simulink model "sampleModel25"  (R2021b)
settings: Solver=VariableStepAuto  StartTime=0.0  StopTime=10.0  RelTol=1e-3
undefined symbols (not defined in the file or in its folder): DiscIntNeverNeededParam, Newton, Raphson
libraries: simulink x8, slpidlib x1
settings Model: Creator=user  LastModifiedBy=user

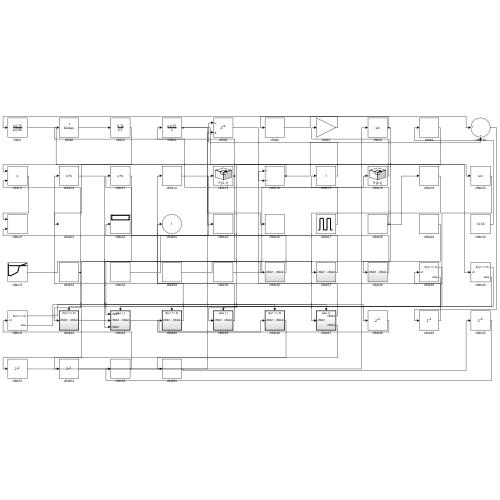
[thumbnail: Simulink's stored preview of the top-level diagram]
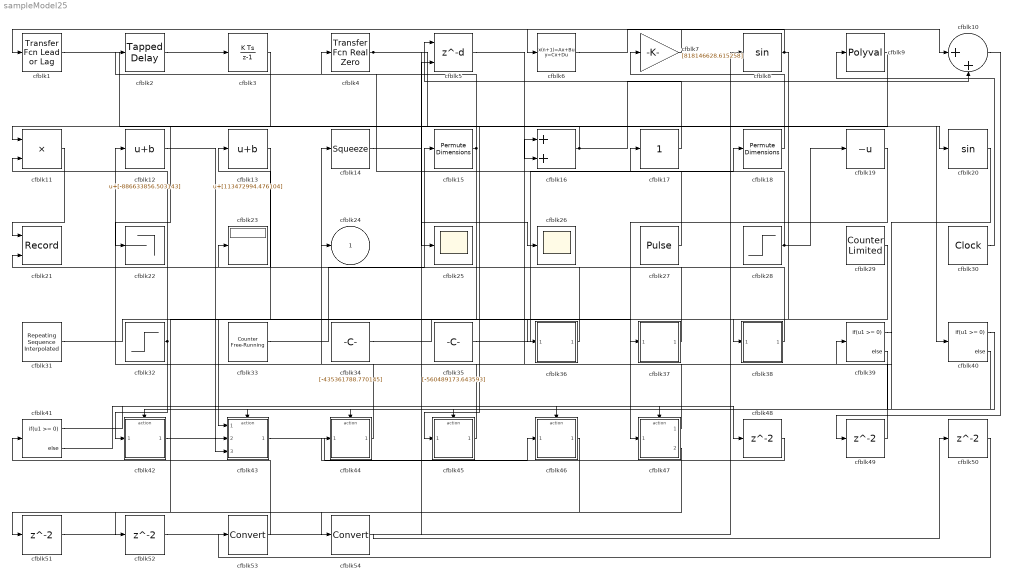
== system sampleModel25 ==
  cfblk1 : simulink/Discrete/Transfer Fcn Lead or Lag  PoleZ=0.95  ZeroZ=0.75  ICPrevOutput=0.0  ICPrevInput=0.0  DoSatur=off
      settings: SourceProductBaseCode=SL
  cfblk10 : Sum  Inputs=|++
  cfblk11 : Product  Inputs=**
  cfblk12 : Bias  Bias=[-886633856.503143]
  cfblk13 : Bias  Bias=[113472994.476104]
  cfblk14 : Squeeze
  cfblk15 : PermuteDimensions
  cfblk16 : Sum
  cfblk17 : simulink/Math Operations/Slider Gain  gain=1  low=0  high=2
  cfblk18 : PermuteDimensions
  cfblk19 : UnaryMinus
  cfblk2 : simulink/Discrete/Tapped Delay  vinit=0.0  samptime=-1  NumDelays=1  DelayOrder=Oldest  includeCurrent=off
  cfblk20 : Trigonometry
  cfblk21 : Record  FileSettingsInternal="{\"entries\":[{\"content\":{\"excelSettings\":{\"content\":{},\"type\":\"Streamout.ExcelSettings\"}},\"type\":\"Streamout.FileSettingStorage\",\"uuid\":\"81ea7c7e-9fea-4c93-8eb7-3e8b3ac382b8\"}],\"packageUris\":[\"http://schema.mathworks.com/mf0/streamout_blocks/R2020a\"],\"version\":\"1.0\"}"  Layout=[1 1]  SignalsInternal="{\"entries\":[{\"content\":{\"signals\":[{\"content\":{\"blockPath\":[\"sampleModel25/cfblk21\"],\"channel\":[],\"dimensions\":[1],\"domain\":\"sampleModel25/cfblk21\",\"lineColor\":\"#a2142f\",\"plots\":[1],\"port\":1,\"sid\":[\"\"],\"signalID\":958,\"signalName\":\"cfblk11\"},\"type\":\"RecordBlkView.Signal\",\"uuid\":\"227c1af8-843d-4dbb-83c8-0e7a03416cd8\"},{\"content\":{\"blockPath\":[\"sampleModel25/cfblk21\"],\"channel\":[],\"dimensions\":[1],\"domain\":\"sampleModel25/cfblk21\",\"lineColor\":\"#139fff\",\"plots\":[1],\"port\":2,\"sid\":[\"\"],\"signalID\":962,\"signalName\":\"cfblk36\"},\"type\":\"RecordBlkView.Signal\",\"uuid\":\"4e12becd-70fb-4f71-8634-a0132a2030ff\"}]},\"type\":\"RecordBlkView.InputSignals\",\"uuid\":\"b961e02f-62d7-4da1-8324-0dc8cbebac20\"}],\"packageUris\":[\"http://schema.mathworks.com/mf0/streamout_blocks/R2020a\"],\"version\":\"1.0\"}"  VisualizationBindings="{\"xyplotplugin\":{\"info\":[{\"series\":[{\"bindingParametersList\":[{\"parameter\":\"X-Axis\",\"signalID\":958,\"signalName\":\"cfblk11\"},{\"parameter\":\"Y-Axis\",\"signalID\":962,\"signalName\":\"cfblk36\"}],\"seriesID\":47306}],\"subplotID\":1}]}}"  CompatibilityTag=XY
  cfblk22 : Terminator
  cfblk23 : Display
  cfblk25 : Scope
  cfblk26 : Scope
  cfblk27 : DiscretePulseGenerator  PulseType=Time based  Amplitude=[-185017419.395854]  Period=[23344587.836266]  PulseWidth=5  PhaseDelay=[5.000000]
  cfblk28 : Step  Time=[16.000000]  Before=[417268794.168945]  After=[174121089.074614]  SampleTime=0
  cfblk29 : simulink/Sources/Counter Limited  uplimit=[239.000000]  tsamp=-1
  cfblk3 : DiscreteIntegrator  ICPrevOutput=DiscIntNeverNeededParam  ICPrevScaledInput=DiscIntNeverNeededParam
  cfblk30 : DigitalClock
  cfblk31 : simulink/Sources/Repeating Sequence Interpolated  OutValues=[-871882158.098314, -993261613.147159, -621854313.016368, -17592622.938083, 232937701.934326]  TimeValues=[0 0.1 0.5 0.6 1].'  LookUpMeth=Interpolation-Use End Values  tsamp=0.01  OutMin=[]  OutMax=[]  OutDataTypeStr=double  OutputDataTypeScalingMode=double  OutDataType=fixdt(0,8)  OutScaling=2^-10
  cfblk32 : Step  Time=[7.000000]  Before=[-371638337.003964]  After=[-824289697.887476]  SampleTime=0
  cfblk33 : simulink/Sources/Counter Free-Running  NumBits=[25.000000]  tsamp=-1
  cfblk34 : Constant  Value=[-435361788.770145]  SampleTime=1
  cfblk35 : Constant  Value=[-560489173.643593]  SampleTime=1
  cfblk36 : Subsystem
  cfblk37 : Subsystem
  cfblk38 : Subsystem
  cfblk39 : If  IfExpression=u1 >= 0  SampleTime=1
  cfblk4 : simulink/Discrete/Transfer Fcn Real Zero  ZeroZ=0.75  ICPrevInput=0.0  DoSatur=off
      settings: SourceProductBaseCode=SL
  cfblk40 : If  IfExpression=u1 >= 0  SampleTime=1
  cfblk41 : If  IfExpression=u1 >= 0  SampleTime=1
  cfblk42 : Subsystem  TreatAsAtomicUnit=on
  cfblk43 : Subsystem  TreatAsAtomicUnit=on
  cfblk44 : Subsystem  TreatAsAtomicUnit=on
  cfblk45 : Subsystem  TreatAsAtomicUnit=on
  cfblk46 : Subsystem  TreatAsAtomicUnit=on
  cfblk47 : Subsystem  TreatAsAtomicUnit=on
  cfblk{48..52} (5 alike) : Delay  SampleTime=1
  cfblk5 : Delay  DelayLengthSource=Input port  SampleTime=1
      settings: InputPortMap=u0,p1
  cfblk53 : DataTypeConversion
  cfblk54 : DataTypeConversion
  cfblk6 : DiscreteStateSpace
  cfblk7 : Gain  Gain=[818146628.615258]
  cfblk8 : Trigonometry
  cfblk9 : Polyval  Coefs=[ +2.081618890e-019, -1.441693666e-014, +4.719686976e-010, -8.536869453e-006, +1.621573104e-001, -8.087801117e+001 ]
  cfblk24 : Outport
  wires:
  cfblk29/1 -> cfblk43/1(cfblk1)
  cfblk32/1 -> cfblk42/1(cfblk1), cfblk11/2
  cfblk20/1 -> cfblk39/1
  cfblk8/1 -> cfblk1/1, cfblk38/1(cfblk1)
  cfblk28/1 -> cfblk17/1, cfblk19/1
  cfblk33/1 -> cfblk15/1
  cfblk37/1(cfblk2) -> cfblk23/1
  cfblk18/1 -> cfblk7/1
  cfblk47/1(cfblk2) -> cfblk14/1
  cfblk43/1(cfblk2) -> cfblk46/1(cfblk1)
  cfblk35/1 -> cfblk18/1
  cfblk17/1 -> cfblk5/1
  cfblk44/1(cfblk2) -> cfblk12/1
  cfblk7/1 -> cfblk6/1
  cfblk3/1 -> cfblk22/1
  cfblk30/1 -> cfblk9/1
  cfblk27/1 -> cfblk4/1
  cfblk15/1 -> cfblk43/2(cfblk4), cfblk2/1
  cfblk38/1(cfblk2) -> cfblk13/1
  cfblk19/1 -> cfblk47/1(cfblk1)
  cfblk11/1 -> cfblk21/1
  cfblk45/1(cfblk2) -> cfblk24/1
  cfblk31/1 -> cfblk37/1(cfblk1)
  cfblk2/1 -> cfblk3/1
  cfblk14/1 -> cfblk26/1
  cfblk1/1 -> cfblk25/1
  cfblk34/1 -> cfblk36/1(cfblk1)
  cfblk5/1 -> cfblk20/1
  cfblk16/1 -> cfblk11/1, cfblk10/2
  cfblk6/1 -> cfblk10/1
  cfblk4/1 -> cfblk40/1, cfblk16/2
  cfblk36/1(cfblk2) -> cfblk21/2
  cfblk9/1 -> cfblk45/1(cfblk1)
  cfblk42/1(cfblk2) -> cfblk43/3(cfblk5)
  cfblk39/1 -> cfblk42/Action
  cfblk39/2 -> cfblk43/Action
  cfblk40/1 -> cfblk44/Action
  cfblk40/2 -> cfblk45/Action
  cfblk41/1 -> cfblk46/Action
  cfblk41/2 -> cfblk47/Action
  cfblk12/1 -> cfblk48/1
  cfblk48/1 -> cfblk44/1(cfblk1)
  cfblk10/1 -> cfblk49/1
  cfblk49/1 -> cfblk16/1
  cfblk47/2(cfblk4) -> cfblk51/1
  cfblk51/1 -> cfblk5/2
  cfblk13/1 -> cfblk52/1
  cfblk52/1 -> cfblk8/1
  cfblk50/1 -> cfblk53/1
  cfblk53/1 -> cfblk41/1
  cfblk46/1(cfblk2) -> cfblk54/1
  cfblk54/1 -> cfblk50/1

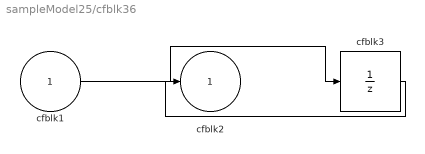
== system sampleModel25/cfblk36 ==
  cfblk1 : Inport
  cfblk3 : UnitDelay  HasFrameUpgradeWarning=on
  cfblk2 : Outport
  wires:
  cfblk1/1 -> cfblk3/1
  cfblk3/1 -> cfblk2/1

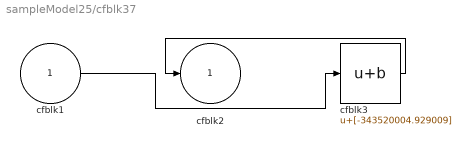
== system sampleModel25/cfblk37 ==
  cfblk1 : Inport
  cfblk3 : Bias  Bias=[-343520004.929009]
  cfblk2 : Outport
  wires:
  cfblk3/1 -> cfblk2/1
  cfblk1/1 -> cfblk3/1

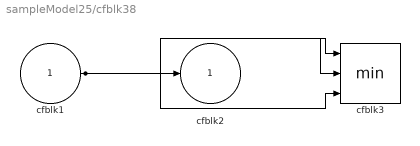
== system sampleModel25/cfblk38 ==
  cfblk1 : Inport
  cfblk3 : MinMax  Inputs=3
  cfblk2 : Outport
  wires:
  cfblk1/1 -> cfblk2/1, cfblk3/1, cfblk3/2, cfblk3/3

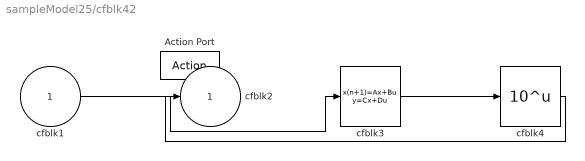
== system sampleModel25/cfblk42 ==
  cfblk1 : Inport
  Action Port : ActionPort  ActionPortLabel=if(u1 >= 0)
  cfblk3 : DiscreteStateSpace  SampleTime=-1
  cfblk4 : Math  Operator=10^u  SaturateOnIntegerOverflow=on
  cfblk2 : Outport
  wires:
  cfblk1/1 -> cfblk3/1
  cfblk3/1 -> cfblk4/1
  cfblk4/1 -> cfblk2/1

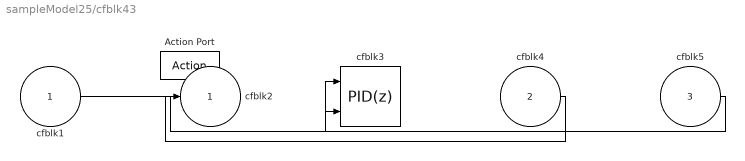
== system sampleModel25/cfblk43 ==
  cfblk1 : Inport
  cfblk4 : Inport  Port=2
  cfblk5 : Inport  Port=3
  Action Port : ActionPort  ActionPortLabel=else
  cfblk3 : slpidlib/PID Controller (2DOF)  Controller=PID  Form=Parallel  TimeDomain=Discrete-time  UseExternalTs=off  SampleTime=-1  IntegratorMethod=Forward Euler  FilterMethod=Forward Euler  ControllerParametersSource=internal  P=1  I=1  D=0  UseFilter=on  N=100  b=1  c=1  TunerSelectOption=Transfer Function Based (PID Tuner App)  InitialConditionSource=internal  InitialConditionForIntegrator=0  InitialConditionForFilter=0  DifferentiatorICPrevScaledInput=0  ExternalReset=none  TrackingMode=off  Kt=1  LimitOutput=off  SatLimitsSource=internal  UpperSaturationLimit=inf  LowerSaturationLimit=-inf  LinearizeAsGain=off  AntiWindupMode=none  Kb=1  POutMin=[]  POutMax=[]  IOutMin=[]  IOutMax=[]  DOutMin=[]  DOutMax=[]  NOutMin=[]  NOutMax=[]  bOutMin=[]  bOutMax=[]  cOutMin=[]  cOutMax=[]  SumOutMin=[]  SumOutMax=[]  SaturationOutMin=[]  SaturationOutMax=[]  PParamMin=[]  PParamMax=[]  IParamMin=[]  IParamMax=[]  DParamMin=[]  DParamMax=[]  NParamMin=[]  NParamMax=[]  bParamMin=[]  bParamMax=[]  cParamMin=[]  cParamMax=[]  KbParamMin=[]  KbParamMax=[]  KtParamMin=[]  KtParamMax=[]  KbOutMin=[]  KbOutMax=[]  KtOutMin=[]  KtOutMax=[]  IntegratorOutMin=[]  IntegratorOutMax=[]  FilterOutMin=[]  FilterOutMax=[]  SumI1OutMin=[]  SumI1OutMax=[]  SumI2OutMin=[]  SumI2OutMax=[]  SumI3OutMin=[]  SumI3OutMax=[]  SumI4OutMin=[]  SumI4OutMax=[]  SumDOutMin=[]  SumDOutMax=[]  Sum1OutMin=[]  Sum1OutMax=[]  Sum2OutMin=[]  Sum2OutMax=[]  Sum3OutMin=[]  Sum3OutMax=[]  DifferentiatorOutMin=[]  DifferentiatorOutMax=[]  FilterDiffOutCoefMin=[]  FilterDiffOutCoefMax=[]  ReciprocalOutMin=[]  ReciprocalOutMax=[]  SumDenOutMin=[]  SumDenOutMax=[]  SumNumOutMin=[]  SumNumOutMax=[]  DivideOutMin=[]  DivideOutMax=[]  UdiffTsProdOutMin=[]  UdiffTsProdOutMax=[]  NTsProdOutMin=[]  NTsProdOutMax=[]  UintegralTsProdOutMin=[]  UintegralTsProdOutMax=[]  UngainTsProdOutMin=[]  UngainTsProdOutMax=[]  IntegratorContinuousStateAttributes=''  IntegratorStateMustResolveToSignalObject=off  IntegratorRTWStateStorageClass=Auto  FilterContinuousStateAttributes=''  FilterStateMustResolveToSignalObject=off  FilterRTWStateStorageClass=Auto  ParallelPVariant=InternalParameters  IdealPVariant=Disabled  IVariant=InternalParameters  DVariant=InternalParameters  bVariant=InternalParameters  cVariant=InternalParameters  IntegratorVariant=Discrete  SatVariant=Disabled  AWVariant=Passthrough  PCopyVariant=Disabled  TRVariant=Disabled  FdbkBlocksVariant=Forward  IdealPFdbkVariant=Disabled  SatFdbkVariant=Disabled  DerivativeFilterVariant=ForwardEulerFilter  NVariant=InternalParameters  NCopyVariant=Disabled  FilterICVariant=InternalICsFilter  IntegratorICVariant=InternalICs  ExternalResetVariant=Disabled  TRSumVariant=Passthrough  SumFdbkVariant=Disabled  SumVariant=Sum_PID  TsampFilterVariant=InternalTs  TsampNgainVariant=Passthrough  TsampIntegralVariant=Passthrough  ExternalSaturationOutDataTypeStr=Inherit: Same as second input
      settings: SourceProductBaseCode=SL
  cfblk2 : Outport
  wires:
  cfblk1/1 -> cfblk3/1
  cfblk4/1 -> cfblk2/1
  cfblk5/1 -> cfblk3/2

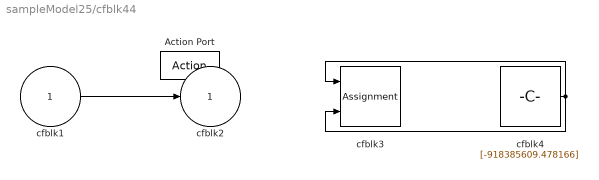
== system sampleModel25/cfblk44 ==
  cfblk1 : Inport
  Action Port : ActionPort  ActionPortLabel=if(u1 >= 0)
  cfblk3 : Assignment  DiagnosticForDimensions=Warning  IndexOptions=Index vector (dialog)  Indices=1  OutputSizes=1
  cfblk4 : Constant  Value=[-918385609.478166]  SampleTime=1
  cfblk2 : Outport
  wires:
  cfblk1/1 -> cfblk2/1
  cfblk4/1 -> cfblk3/1, cfblk3/2

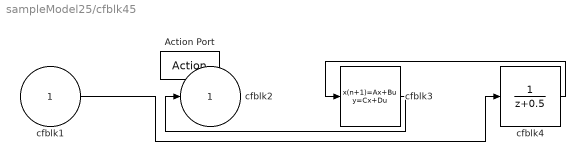
== system sampleModel25/cfblk45 ==
  cfblk1 : Inport
  Action Port : ActionPort  ActionPortLabel=else
  cfblk3 : DiscreteStateSpace  SampleTime=-1
  cfblk4 : DiscreteTransferFcn
  cfblk2 : Outport
  wires:
  cfblk3/1 -> cfblk2/1
  cfblk1/1 -> cfblk4/1
  cfblk4/1 -> cfblk3/1

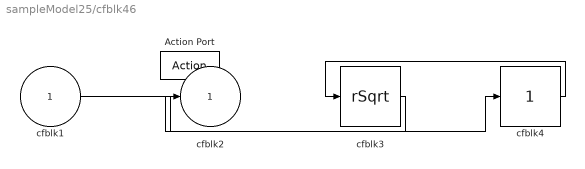
== system sampleModel25/cfblk46 ==
  cfblk1 : Inport
  Action Port : ActionPort  ActionPortLabel=if(u1 >= 0)
  cfblk3 : Sqrt  Operator=rSqrt  AlgorithmType=Newton-Raphson  SaturateOnIntegerOverflow=on
  cfblk4 : simulink/Math Operations/Slider Gain  gain=1  low=0  high=2
  cfblk2 : Outport
  wires:
  cfblk1/1 -> cfblk4/1
  cfblk4/1 -> cfblk3/1
  cfblk3/1 -> cfblk2/1

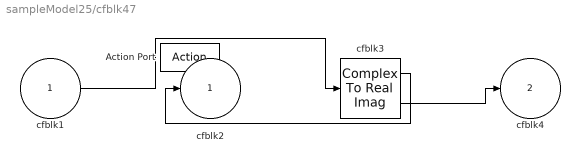
== system sampleModel25/cfblk47 ==
  cfblk1 : Inport
  Action Port : ActionPort  ActionPortLabel=else
  cfblk3 : ComplexToRealImag
  cfblk2 : Outport
  cfblk4 : Outport  Port=2
  wires:
  cfblk3/1 -> cfblk2/1
  cfblk1/1 -> cfblk3/1
  cfblk3/2 -> cfblk4/1
